simulink model "mech_conveyor_vr"  (Simulink 6.0)
settings: Solver=ode45  StartTime=0  StopTime=inf  FixedStep=0.1  RelTol=1e-4  AbsTol=1e-6
PreLoadFcn:
  | load mech_conveyor_controller;
InitFcn:
  | mech_slider_open('mech_conveyor_vr')
undefined symbols (not defined in the file or in its folder): Ak, Aw, Awinv, Bk, Bw, Bwinv, Ck, Cw, Cwinv, Dk, Dw, Dwinv
libraries: mblibv1 x27, simulink x1, vrlib x1
settings Model: Creator=arnav  LastModifiedBy=batserve  ExtModeAutoUpdateStatusClock=off
settings DataIOCC: SignalLoggingName=sigsOut
settings OptimizationCC: BooleanDataType=off  InlineInvariantSignals=off
settings DebuggingCC: AlgebraicLoopMsg=none  CheckExecutionContextPreStartOutputMsg=on  CheckExecutionContextRuntimeOutputMsg=on  SolverPrmCheckMsg=none  UnconnectedInputMsg=none  UnconnectedOutputMsg=none  UnconnectedLineMsg=none
settings HardwareCC: TargetUnknown=on
settings SimMechanicsCC: WarnOnRedundantConstraints=off

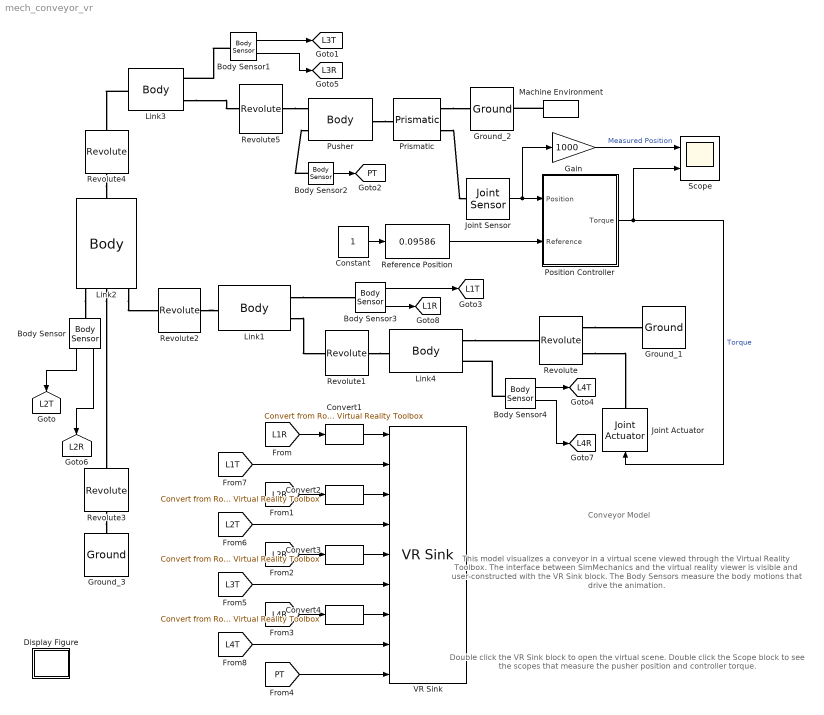
== system mech_conveyor_vr ==
  note: Conveyor Model
  note: This model visualizes a conveyor in a virtual scene
      | viewed through the Virtual Reality Toolbox.  The
      | interface between SimMechanics and the virtual
      | reality viewer is visible and user-constructed with
      | the VR Sink block.  The Body Sensors measure
      | the body motions that drive the animation.
  note: Double click the VR Sink block to open
      | the virtual scene.  Double click
      | the Scope block to see the scopes that measure
      | the pusher position and controller torque.
  Body Sensor : mblibv1/Sensors &  Actuators/Body Sensor  Description=Mechanical Blockset  Orientation=down  Opaque=on  PhysicalDomain=Mechanical  PortType=blob  Muxed=off  Pose=on  Angle=on  AngleUnits=deg  ArcVelocity=off  ArcVelocityUnits=deg/s  ArcAcceleration=off  ArcAccelerationUnits=deg/s^2  CoordPosition=on  CoordPositionUnits=m  Velocity=off  VelocityUnits=m/s  Acceleration=off  AccelerationUnits=m/s^2  Quaternion=on  QuaternionDT=off  QuaternionDDT=off  QuaternionUnits=off  OutputVector=[ 3 9 ]  ActiveIO=on  Width=12  DialogClass=MechanicalSensorBlock  ReferenceFrame=Absolute (World)
  Body Sensor1 : mblibv1/Sensors &  Actuators/Body Sensor  Description=Mechanical Blockset  Opaque=on  PhysicalDomain=Mechanical  PortType=blob  Muxed=off  Pose=on  Angle=on  AngleUnits=deg  ArcVelocity=off  ArcVelocityUnits=deg/s  ArcAcceleration=off  ArcAccelerationUnits=deg/s^2  CoordPosition=on  CoordPositionUnits=m  Velocity=off  VelocityUnits=m/s  Acceleration=off  AccelerationUnits=m/s^2  Quaternion=on  QuaternionDT=off  QuaternionDDT=off  QuaternionUnits=off  OutputVector=[ 3 9 ]  ActiveIO=on  Width=12  DialogClass=MechanicalSensorBlock  ReferenceFrame=Absolute (World)
  Body Sensor2 : mblibv1/Sensors &  Actuators/Body Sensor  Description=Mechanical Blockset  Opaque=on  PhysicalDomain=Mechanical  PortType=blob  Muxed=on  Pose=off  Angle=on  AngleUnits=deg  ArcVelocity=off  ArcVelocityUnits=deg/s  ArcAcceleration=off  ArcAccelerationUnits=deg/s^2  CoordPosition=on  CoordPositionUnits=m  Velocity=off  VelocityUnits=m/s  Acceleration=off  AccelerationUnits=m/s^2  Quaternion=on  QuaternionDT=off  QuaternionDDT=off  QuaternionUnits=off  OutputVector=[ 3 ]  ActiveIO=on  Width=3  DialogClass=MechanicalSensorBlock  ReferenceFrame=Absolute (World)
  Body Sensor3 : mblibv1/Sensors &  Actuators/Body Sensor  Description=Mechanical Blockset  Opaque=on  PhysicalDomain=Mechanical  PortType=blob  Muxed=off  Pose=on  Angle=on  AngleUnits=deg  ArcVelocity=off  ArcVelocityUnits=deg/s  ArcAcceleration=off  ArcAccelerationUnits=deg/s^2  CoordPosition=on  CoordPositionUnits=m  Velocity=off  VelocityUnits=m/s  Acceleration=off  AccelerationUnits=m/s^2  Quaternion=on  QuaternionDT=off  QuaternionDDT=off  QuaternionUnits=off  OutputVector=[ 3 9 ]  ActiveIO=on  Width=12  DialogClass=MechanicalSensorBlock  ReferenceFrame=Absolute (World)
  Body Sensor4 : mblibv1/Sensors &  Actuators/Body Sensor  Description=Mechanical Blockset  Opaque=on  PhysicalDomain=Mechanical  PortType=blob  Muxed=off  Pose=on  Angle=on  AngleUnits=deg  ArcVelocity=off  ArcVelocityUnits=deg/s  ArcAcceleration=off  ArcAccelerationUnits=deg/s^2  CoordPosition=on  CoordPositionUnits=m  Velocity=off  VelocityUnits=m/s  Acceleration=off  AccelerationUnits=m/s^2  Quaternion=on  QuaternionDT=off  QuaternionDDT=off  QuaternionUnits=off  OutputVector=[ 3 9 ]  ActiveIO=on  Width=12  DialogClass=MechanicalSensorBlock  ReferenceFrame=Absolute (World)
  Constant : Constant
  Convert{1..4} (4 alike) : mblibv1/Utilities/Convert from Rotation Matrix to Virtual Reality Toolbox  Tag=Pose2VR
  Display Figure : Subsystem  Tag=Help  Description="Help callback for virtual reality conveyor model: mech_conveyor_vr.  Opens Help browser to Type 19 marker at documentation for this tutorial model."
      settings: AttributesFormatString=\n\n\n  OpenFcn=helpview([docroot '/toolbox/physmod/mech/mech.map'], 'mech_conveyor_vr_help');
      mask Type: Help callback
      mask Display: disp('?');
  Gain : Gain  Gain=1000  SaturateOnIntegerOverflow=on
  Ground_1 : mblibv1/Bodies/Ground  Orientation=left  Opaque=on  LeftPortType=env  RightPortType=workingframe  PhysicalDomain=Mechanical  DialogClass=GroundBlock  CoordPosition=[0.280 0.210 0]  CoordPositionUnits=m  StateVectorMgrId=-1  MachineId=[0 0]  ShowEnvPort=off
  Ground_2 : mblibv1/Bodies/Ground  Orientation=left  Opaque=on  LeftPortType=env  RightPortType=workingframe  PhysicalDomain=Mechanical  DialogClass=GroundBlock  CoordPosition=[0.412 0.5 0]  CoordPositionUnits=m  StateVectorMgrId=-1  MachineId=[0 0]  ShowEnvPort=on
  Ground_3 : mblibv1/Bodies/Ground  Orientation=up  Opaque=on  LeftPortType=env  RightPortType=workingframe  PhysicalDomain=Mechanical  DialogClass=GroundBlock  CoordPosition=[0.08 0.11 0]  CoordPositionUnits=m  StateVectorMgrId=-1  MachineId=[0 0]  ShowEnvPort=off
  Joint Actuator : mblibv1/Sensors &  Actuators/Joint Actuator  Description=Mechanical Blockset  Orientation=up  Opaque=on  PhysicalDomain=Mechanical  PortType=blob  ActuationStyle=Force  AngleUnits=rad  ArcVelocityUnits=rad/s  ArcAccelerationUnits=rad/s^2  CoordPositionUnits=m  VelocityUnits=m/s  AccelerationUnits=m/s^2  ForceUnits=N  TorqueUnits=N-m  ActiveIO=on  Width=1  DialogClass=MechanicalActuatorBlock  Primitive=R1  ReferenceFrame=Absolute (INERTIAL)
  Joint Sensor : mblibv1/Sensors &  Actuators/Joint Sensor  Description=Mechanical Blockset  Opaque=on  PhysicalDomain=Mechanical  PortType=blob  Muxed=on  Pose=off  Angle=on  AngleUnits=deg  ArcVelocity=off  ArcVelocityUnits=deg/s  ArcAcceleration=off  ArcAccelerationUnits=deg/s^2  CoordPosition=on  CoordPositionUnits=m  Velocity=off  VelocityUnits=m/s  Acceleration=off  AccelerationUnits=m/s^2  Quaternion=on  QuaternionDT=off  QuaternionDDT=off  QuaternionUnits=off  OutputVector=[ 1 ]  ActiveIO=on  Width=1  DialogClass=MechanicalSensorBlock  Primitive=P1  Force=off  ForceUnits=N  Torque=off  TorqueUnits=N-m  ReferenceFrame=Absolute (INERTIAL)  ReactionSensedSide=Base  ReactionReferenceFrame=Absolute (World)  ReactionForce=off  ReactionForceUnits=N  ReactionMoment=off  ReactionMomentUnits=N-m
  Link1 : mblibv1/Bodies/Body  Tag=Factory generic  Description=Mechanical Blockset  Orientation=left  PhysicalDomain=mechanical  SubClassName=Unknown  LeftPortType=workingframe  RightPortType=workingframe  LConnTagsString=CS3|CS1  RConnTagsString=CS2  DialogClass=MechanicalBodyBlock  Mass=0.98785  MassUnits=kg  InertiaUnits=kg*m^2  Inertia=[7.6414e-005 -9.2222e-005 1.8971e-009;-9.2222e-005 0.0083286 -2.5235e-010;1.8971e-009 -2.5235e-010 0.0083397]  Shape=Cylinder  ShapeDims=[1 1]  ShapeUnits=m  ShapeUse=false  Density=1  DensityUnits=kg/m^3  DensityUse=false  CG=Left$CG$[0.110 0.247 0]$WORLD$WORLD$m$[0 0 -4.22]$Euler X-Y-Z$deg$WORLD$false  WorkingFrames=Left$CS3$[0 0 0]$WORLD$WORLD$m$[0 0 0]$Euler X-Y-Z$deg$WORLD$true#Left$CS1$[0.265 0.236 0]$WORLD$WORLD$m$[0 0 0]$Euler X-Y-Z$deg$WORLD$true#Right$CS2$[-0.299 0.022 0]$WORLD$CS1$m$[0 0 0]$Euler X-Y-Z$deg$WORLD$true
  Link2 : mblibv1/Bodies/Body  Tag=Factory generic  Description=Mechanical Blockset  Orientation=up  PhysicalDomain=mechanical  SubClassName=Unknown  LeftPortType=workingframe  RightPortType=workingframe  LConnTagsString=CS4|CS1|CS2  RConnTagsString=CS3  DialogClass=MechanicalBodyBlock  Mass=2.7433  MassUnits=kg  InertiaUnits=kg*m^2  Inertia=[0.0044915 2.9472e-005 1.0996e-007;2.9472e-005 0.089001 -4.3534e-007;1.0996e-007 -4.3534e-007 0.093312]  Shape=Cylinder  ShapeDims=[1 1]  ShapeUnits=m  ShapeUse=false  Density=1  DensityUnits=kg/m^3  DensityUse=false  CG=Left$CG$[-0.030 0.402 0]$WORLD$WORLD$m$[0 0 95.31]$Euler X-Y-Z$deg$WORLD$false  WorkingFrames=Left$CS4$[0 0 0]$WORLD$WORLD$m$[0 0 0]$Euler X-Y-Z$deg$WORLD$true#Left$CS1$[0.08 0.11 0]$WORLD$WORLD$m$[0 0 0]$Euler X-Y-Z$deg$WORLD$true#Left$CS2$[-0.114 0.148 0]$WORLD$CS1$m$[0 0 0]$Euler X-Y-Z$deg$WORLD$true#Right$CS3$[0.059 0.449 0]$WORLD$CS2$m$[0 0 0]$Euler X-Y-Z$deg$WORLD$true
  Link3 : mblibv1/Bodies/Body  Tag=Factory generic  Description=Mechanical Blockset  PhysicalDomain=mechanical  SubClassName=Unknown  LeftPortType=workingframe  RightPortType=workingframe  LConnTagsString=CS1  RConnTagsString=CS3|CS2  DialogClass=MechanicalBodyBlock  Mass=1.2355  MassUnits=kg  InertiaUnits=kg*m^2  Inertia=[8.2129e-005 1.8216e-005 -3.7069e-010;1.8216e-005 0.017391 -2.6914e-011;-3.7069e-010 -2.6914e-011 0.017392]  Shape=Cylinder  ShapeDims=[1 1]  ShapeUnits=m  ShapeUse=false  Density=1  DensityUnits=kg/m^3  DensityUse=false  CG=Left$CG$[0.194 0.604 0.01]$WORLD$WORLD$m$[90 -31.24 0]$Euler X-Y-Z$deg$WORLD$false  WorkingFrames=Right$CS3$[0 0 0]$WORLD$WORLD$m$[0 0 0]$Euler X-Y-Z$deg$WORLD$true#Left$CS1$[0.025 0.707 0]$WORLD$WORLD$m$[0 0 0]$Euler X-Y-Z$deg$WORLD$true#Right$CS2$[0.342 -0.207 0]$WORLD$CS1$m$[0 0 0]$Euler X-Y-Z$deg$WORLD$true
  Link4 : mblibv1/Bodies/Body  Tag=Factory generic  Description=Mechanical Blockset  Orientation=left  PhysicalDomain=mechanical  SubClassName=Unknown  LeftPortType=workingframe  RightPortType=workingframe  LConnTagsString=CS1|CS3  RConnTagsString=CS2  DialogClass=MechanicalBodyBlock  Mass=0.057538  MassUnits=kg  InertiaUnits=kg*m^2  Inertia=[1.0148e-005 0 0;0 2.5218e-006 0;0 0 1.1711e-005]  Shape=Cylinder  ShapeDims=[1 1]  ShapeUnits=m  ShapeUse=false  Density=1  DensityUnits=kg/m^3  DensityUse=false  CG=Left$CG$[0.272 0.223 0.01]$WORLD$WORLD$m$[0 0 30]$Euler X-Y-Z$deg$WORLD$false  WorkingFrames=Left$CS1$[0.280 0.210 0]$WORLD$WORLD$m$[0 0 0]$Euler X-Y-Z$deg$WORLD$true#Right$CS2$[-0.015 0.026 0]$CS1$CS1$m$[0 0 0]$Euler X-Y-Z$deg$WORLD$true#Left$CS3$[0 0 0]$WORLD$WORLD$m$[0 0 0]$Euler X-Y-Z$deg$WORLD$true
  Machine Environment : mblibv1/Bodies/Machine Environment  Tag=Factory ground  Orientation=left  DialogController=MECH.DialogSource  Opaque=on  PortType=env  PhysicalDomain=Mechanical  DialogTemplateClass=MECH.MachineEnvironment  SyncWhenCopied=off  Gravity=[0 -9.81 0]  GravityUnits=m/s^2  GravityAsSignal=off  Dimensionality=3D Only  AnalysisType=Forward dynamics  LinearAssemblyTolerance=1e-3  LinearAssemblyToleranceUnits=m  AngularAssemblyTolerance=1e-3  AngularAssemblyToleranceUnits=rad  ConstraintSolverType=Stabilizing  ConstraintRelTolerance=1e-4  ConstraintAbsTolerance=1e-4  UseRobustSingularityHandling=off  StatePerturbationType=Adaptive  PerturbationSize=1e-3  VisualizeMachine=on
  Position Controller : Subsystem
  Prismatic : mblibv1/Joints/Prismatic  Tag=Factory generic  Description=Mechanical Blockset  Orientation=left  PhysicalDomain=mechanical  SubClassName=Unknown  LeftPortType=blob  RightPortType=blob  LConnTagsString=__newl0|SA1  RConnTagsString=__newr0  NumSAPorts=1  CutJoint=off  MarkAsCut=off  Primitives=prismatic  PrimitiveProps=P1$WORLD$[1 0 0]$prismatic  DialogClass=JointBlock
  Pusher : mblibv1/Bodies/Body  Tag=Factory generic  Description=Mechanical Blockset  PhysicalDomain=mechanical  SubClassName=Unknown  LeftPortType=workingframe  RightPortType=workingframe  LConnTagsString=CS1|CS3  RConnTagsString=CS2  DialogClass=MechanicalBodyBlock  Mass=1.8547  MassUnits=kg  InertiaUnits=kg*m^2  Inertia=[0.0025031 -1.671e-006 5.5014e-006;-1.671e-006 0.0016406 -1.8596e-007;5.5014e-006 -1.8596e-007 0.0011862]  Shape=Cylinder  ShapeDims=[1 1]  ShapeUnits=m  ShapeUse=false  Density=1  DensityUnits=kg/m^3  DensityUse=false  CG=Left$CG$[0.396 0.499 0]$WORLD$WORLD$m$[0 0 0]$Euler X-Y-Z$deg$WORLD$false  WorkingFrames=Left$CS1$[0.367 0.5 0]$WORLD$WORLD$m$[0 0 0]$Euler X-Y-Z$deg$WORLD$true#Right$CS2$[0.045 0 0]$WORLD$CS1$m$[0 0 0]$Euler X-Y-Z$deg$WORLD$true#Left$CS3$[0 0 0]$WORLD$WORLD$m$[0 0 0]$Euler X-Y-Z$deg$WORLD$true
  Reference Position : simulink/Math Operations/Slider Gain  Tag="685  498  330   98"  low=0  gain=0.09586  high=0.2
  Revolute : mblibv1/Joints/Revolute  Tag=Factory generic  Description=Mechanical Blockset  Orientation=left  PhysicalDomain=mechanical  SubClassName=Unknown  LeftPortType=blob  RightPortType=blob  LConnTagsString=__newl0|SA1  RConnTagsString=__newr0  NumSAPorts=1  CutJoint=off  MarkAsCut=off  Primitives=revolute  PrimitiveProps=R1$WORLD$[0 0 1]$revolute  DialogClass=JointBlock
  Revolute1 : mblibv1/Joints/Revolute  Tag=Factory generic  Description=Mechanical Blockset  Orientation=left  PhysicalDomain=mechanical  SubClassName=Unknown  LeftPortType=blob  RightPortType=blob  LConnTagsString=__newl0  RConnTagsString=__newr0  NumSAPorts=0  CutJoint=off  MarkAsCut=off  Primitives=revolute  PrimitiveProps=R1$WORLD$[0 0 1]$revolute  DialogClass=JointBlock
  Revolute2 : mblibv1/Joints/Revolute  Tag=Factory generic  Description=Mechanical Blockset  Orientation=left  PhysicalDomain=mechanical  SubClassName=Unknown  LeftPortType=blob  RightPortType=blob  LConnTagsString=__newl0  RConnTagsString=__newr0  NumSAPorts=0  CutJoint=on  MarkAsCut=off  Primitives=revolute  PrimitiveProps=R1$WORLD$[0 0 1]$revolute  DialogClass=JointBlock
  Revolute3 : mblibv1/Joints/Revolute  Tag=Factory generic  Description=Mechanical Blockset  Orientation=up  PhysicalDomain=mechanical  SubClassName=Unknown  LeftPortType=blob  RightPortType=blob  LConnTagsString=__newl0  RConnTagsString=__newr0  NumSAPorts=0  CutJoint=off  MarkAsCut=off  Primitives=revolute  PrimitiveProps=R1$WORLD$[0 0 1]$revolute  DialogClass=JointBlock
  Revolute4 : mblibv1/Joints/Revolute  Tag=Factory generic  Description=Mechanical Blockset  Orientation=up  PhysicalDomain=mechanical  SubClassName=Unknown  LeftPortType=blob  RightPortType=blob  LConnTagsString=__newl0  RConnTagsString=__newr0  NumSAPorts=0  CutJoint=on  MarkAsCut=off  Primitives=revolute  PrimitiveProps=R1$WORLD$[0 0 1]$revolute  DialogClass=JointBlock
  Revolute5 : mblibv1/Joints/Revolute  Tag=Factory generic  Description=Mechanical Blockset  PhysicalDomain=mechanical  SubClassName=Unknown  LeftPortType=blob  RightPortType=blob  LConnTagsString=__newl0  RConnTagsString=__newr0  NumSAPorts=0  CutJoint=off  MarkAsCut=off  Primitives=revolute  PrimitiveProps=R1$WORLD$[0 0 1]$revolute  DialogClass=JointBlock
  Scope : Scope  NumInputPorts=2
      settings: TimeRange=20  YMin=-25~-5  YMax=225~5
  VR Sink : vrlib/VR Sink  SampleTime=0.1  ViewEnable=on  RemoteChange=off  RemoteView=off  FieldsWritten=Link1.rotation.4#Link1.translation.3#Link2.rotation.4#Link2.translation.3#Link3.rotation.4#Link3.translation.3#Link4.rotation.4#Link4.translation.3#Pusher.translation.3  WorldFileName=convmech.wrl  WorldDescription=convmech  AutoView=off  FigureProperties={}
  tag scope: L1R=global, L1T=global, L2R=global, L2T=global, L3R=global, L3T=global, L4R=global, L4T=global, PT=global
  wires:
  Joint Sensor/1 -> Position Controller/1(Position), Gain/1
  Constant/1 -> Reference Position/1
  Position Controller/1(Torque) -> Joint Actuator/1, Scope/2  "Torque"
  Reference Position/1 -> Position Controller/2(Reference)
  Gain/1 -> Scope/1  "Measured Position"
  [L1R] -> Convert1/1
  [L2R] -> Convert2/1
  [L3R] -> Convert3/1
  Body Sensor/1 -> [L2T]
  Body Sensor1/1 -> [L3T]
  Body Sensor2/1 -> [PT]
  Body Sensor3/1 -> [L1T]
  Body Sensor4/1 -> [L4T]
  Body Sensor1/2 -> [L3R]
  Body Sensor/2 -> [L2R]
  [L4R] -> Convert4/1
  Body Sensor4/2 -> [L4R]
  Body Sensor3/2 -> [L1R]
  [L1T] -> VR Sink/2
  Convert2/1 -> VR Sink/3
  [L2T] -> VR Sink/4
  Convert3/1 -> VR Sink/5
  [L3T] -> VR Sink/6
  Convert4/1 -> VR Sink/7
  Convert1/1 -> VR Sink/1
  [L4T] -> VR Sink/8
  [PT] -> VR Sink/9
  connections:
  Link2/LConn2 -- Revolute3/RConn1
  Revolute3/LConn1 -- Ground_3/RConn1
  Revolute4/LConn1 -- Link2/RConn1
  Link2/LConn3 -- Revolute2/RConn1
  Link3/LConn1 -- Revolute4/RConn1
  Link3/RConn2 -- Revolute5/LConn1
  Revolute5/RConn1 -- Pusher/LConn1
  Revolute2/LConn1 -- Link1/RConn1
  Revolute1/LConn1 -- Link4/RConn1
  Link4/LConn1 -- Revolute/RConn1
  Revolute/LConn1 -- Ground_1/RConn1
  Prismatic/LConn2 -- Joint Sensor/LConn1
  Prismatic/LConn1 -- Ground_2/RConn1
  Pusher/RConn1 -- Prismatic/RConn1
  Revolute/LConn2 -- Joint Actuator/RConn1
  Link2/LConn1 -- Body Sensor/LConn1
  Body Sensor1/LConn1 -- Link3/RConn1
  Body Sensor2/LConn1 -- Pusher/LConn2
  Body Sensor4/LConn1 -- Link4/LConn2
  Link1/LConn1 -- Body Sensor3/LConn1
  Link1/LConn2 -- Revolute1/RConn1
  Machine Environment/RConn1 -- Ground_2/LConn1

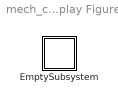
== system mech_conveyor_vr/Display Figure ==
  EmptySubsystem : Subsystem

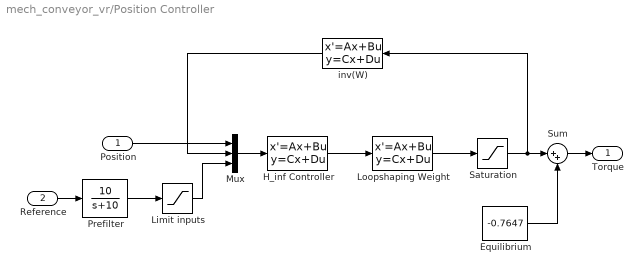
== system mech_conveyor_vr/Position Controller ==
  Position : Inport  Port=1  LatchInput=off
  Reference : Inport  Port=2  LatchInput=off
  Equilibrium : Constant  Value=-0.7647
  H_inf Controller : StateSpace  A=Ak  B=Bk  C=Ck  D=Dk
  Limit inputs : Saturate  UpperLimit=0.2  LowerLimit=0  ZeroCross=off
  Loopshaping Weight : StateSpace  A=Aw  B=Bw  C=Cw  D=Dw
  Mux : Mux  Inputs=3
  Prefilter : TransferFcn  Numerator=[10]  Denominator=[1 10]
  Saturation : Saturate  UpperLimit=5  LowerLimit=-5+0.7647  ZeroCross=off
  Sum : Sum  Inputs=|++  SaturateOnIntegerOverflow=on  InputSameDT=on
  inv(W) : StateSpace  Orientation=left  A=Awinv  B=Bwinv  C=Cwinv  D=Dwinv
  Torque : Outport
  wires:
  H_inf Controller/1 -> Loopshaping Weight/1
  Mux/1 -> H_inf Controller/1
  Position/1 -> Mux/1
  Limit inputs/1 -> Mux/3
  inv(W)/1 -> Mux/2
  Loopshaping Weight/1 -> Saturation/1
  Saturation/1 -> Sum/1, inv(W)/1
  Sum/1 -> Torque/1
  Equilibrium/1 -> Sum/2
  Prefilter/1 -> Limit inputs/1
  Reference/1 -> Prefilter/1

== system mech_conveyor_vr/Display Figure/EmptySubsystem ==
